simulink model "mrefrobotarm_previous_y_previous_u_previous_ref_cex_3b"  (R2018b)
settings: Solver=FixedStepAuto  StartTime=0.0  StopTime=20  RelTol=1e-3  AbsTol=1e-6
undefined symbols (not defined in the file or in its folder): cc, options
libraries: neural x462, simulink x2
(part 4 of 18)

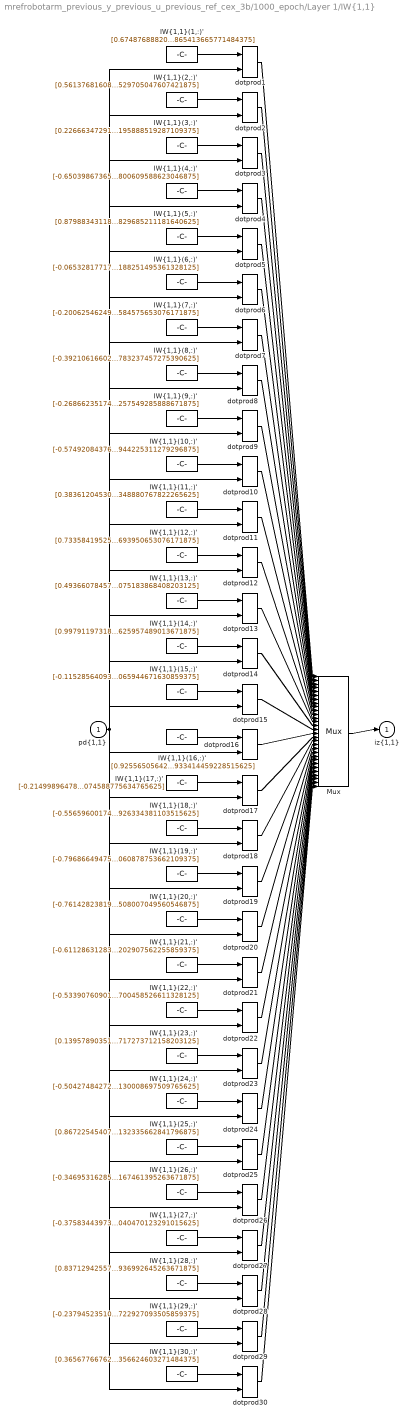
== system mrefrobotarm_previous_y_previous_u_previous_ref_cex_3b/1000_epoch/Layer 1/IW{1,1} ==
  "pd{1,1}" : Inport  PortDimensions=10
      mask Display: e = 0.06;c1 = [120 230 180]/255;c2 = ([120 230 180]+0)/(256+128);c3 = ([120 230 180]+128)/(256+128);patch([0 1 1 0],[0 0 1 1],c1);patch([0 1 1 1-e 1-e 0+e],[0 0 1 1-e 0+e 0+e],c2);patch([0 0 1 1-e 0+e 0+e],[0 1 1 1-e 1-e 0+e],c3);plot([0 1 1 0 0],[0 0 1 1 0]);
  "IW{1,1}(1,:)'" : Constant  Value=[0.67487688820245617105086921583279035985469818115234375;0.489109853240939196350467454976751469075679779052734375;-1.068845446514034680518534514703787863254547119140625;0.21467874123306529554611188359558582305908203125;1.2453232389863388984707626150338910520076751708984375;-0.485155755597752313956760872315499000251293182373046875;0.117400971307613843919170903973281383514404296875;-1.0340884350509644828974842312163673341274261474609375;2.732184740736296912899661037954501807689666748046875;4.26172786638146217086386968730948865413665771484375]
      mask Display: e = 0.06;c1 = [120 150 230]/255;c2 = ([120 150 230]+0)/383;c3 = ([120 150 230]+128)/383;patch([0 1 1 0],[0 0 1 1],c1);patch([0 1 1 1-e 1-e 0+e],[0 0 1 1-e 0+e 0+e],c2);patch([0 0 1 1-e 0+e 0+e],[0 1 1 1-e 1-e 0+e],c3);plot([0 1 1 0 0],[0 0 1 1 0]);disp('Weights');
  "IW{1,1}(10,:)'" : Constant  Value=[-0.57492084376879060148013422804069705307483673095703125;0.11469544369514152182265576129793771542608737945556640625;0.12055448748532505975905593231800594367086887359619140625;-0.55918043406571005249361405731178820133209228515625;-0.95764095097936152711781687685288488864898681640625;-1.877681983780480123868983355350792407989501953125;-4.68369972477810136979314847849309444427490234375;4.12980481084496720001197900273837149143218994140625;-1.55347300362387930050545037374831736087799072265625;-0.04197009317386261872950825591033208183944225311279296875]
      mask Display: e = 0.06;c1 = [120 150 230]/255;c2 = ([120 150 230]+0)/383;c3 = ([120 150 230]+128)/383;patch([0 1 1 0],[0 0 1 1],c1);patch([0 1 1 1-e 1-e 0+e],[0 0 1 1-e 0+e 0+e],c2);patch([0 0 1 1-e 0+e 0+e],[0 1 1 1-e 1-e 0+e],c3);plot([0 1 1 0 0],[0 0 1 1 0]);disp('Weights');
  "IW{1,1}(11,:)'" : Constant  Value=[0.383612045304692339531271727537387050688266754150390625;-0.37441834744799884493460240264539606869220733642578125;-1.572196829190865674519272943143732845783233642578125;-0.469582275713535557404298970141098834574222564697265625;-0.85236355280953490787254622773616574704647064208984375;-0.12317165432347110254340805113315582275390625;0.2987108481842801754879701547906734049320220947265625;0.52483270557119798827017120856908150017261505126953125;0.21737502294189947615876690178993158042430877685546875;0.69653814069038111345122388229356147348880767822265625]
      mask Display: e = 0.06;c1 = [120 150 230]/255;c2 = ([120 150 230]+0)/383;c3 = ([120 150 230]+128)/383;patch([0 1 1 0],[0 0 1 1],c1);patch([0 1 1 1-e 1-e 0+e],[0 0 1 1-e 0+e 0+e],c2);patch([0 0 1 1-e 0+e 0+e],[0 1 1 1-e 1-e 0+e],c3);plot([0 1 1 0 0],[0 0 1 1 0]);disp('Weights');
  "IW{1,1}(12,:)'" : Constant  Value=[0.73358419525220963652856198677909560501575469970703125;0.11073483182108510847196924942181794904172420501708984375;0.239998610252308453016922840106417424976825714111328125;1.3263748611689971657057185439043678343296051025390625;-0.383552641862259402483203984957071952521800994873046875;-0.64895639280684225269624221255071461200714111328125;0.406664060328740972760641625427524559199810028076171875;0.10576433377067527563664128820164478383958339691162109375;-0.1725196998259027891808869981105090118944644927978515625;0.86566960908073908864679424368659965693950653076171875]
      mask Display: e = 0.06;c1 = [120 150 230]/255;c2 = ([120 150 230]+0)/383;c3 = ([120 150 230]+128)/383;patch([0 1 1 0],[0 0 1 1],c1);patch([0 1 1 1-e 1-e 0+e],[0 0 1 1-e 0+e 0+e],c2);patch([0 0 1 1-e 0+e 0+e],[0 1 1 1-e 1-e 0+e],c3);plot([0 1 1 0 0],[0 0 1 1 0]);disp('Weights');
  "IW{1,1}(13,:)'" : Constant  Value=[0.493660784573921096463067215154296718537807464599609375;-0.252852678422424370641152790994965471327304840087890625;0.77470538036599745357335677908849902451038360595703125;0.00925012421792863193115152853351901285350322723388671875;0.93836282792411085384998159497627057135105133056640625;-0.52546190119467095502869824485969729721546173095703125;0.247546801452324161108009548115660436451435089111328125;-0.339457032170829953177104698625043965876102447509765625;-2.052837829371420230728517708485014736652374267578125;-0.70155465814033857174791819488746114075183868408203125]
      mask Display: e = 0.06;c1 = [120 150 230]/255;c2 = ([120 150 230]+0)/383;c3 = ([120 150 230]+128)/383;patch([0 1 1 0],[0 0 1 1],c1);patch([0 1 1 1-e 1-e 0+e],[0 0 1 1-e 0+e 0+e],c2);patch([0 0 1 1-e 0+e 0+e],[0 1 1 1-e 1-e 0+e],c3);plot([0 1 1 0 0],[0 0 1 1 0]);disp('Weights');
  "IW{1,1}(14,:)'" : Constant  Value=[0.99791197318916469161109716878854669630527496337890625;-0.9694834789619761750145698897540569305419921875;-0.341004964206196969911388805485330522060394287109375;1.132787313027051379066278968821279704570770263671875;-0.272808823384909970855005667544901371002197265625;0.283901890384503807762683891269261948764324188232421875;0.57081006863483085833621544225024990737438201904296875;-0.2053654400897696186145680030676885508000850677490234375;-0.1163006140612069250206417336812592111527919769287109375;0.2464533721904866581109416756589780561625957489013671875]
      mask Display: e = 0.06;c1 = [120 150 230]/255;c2 = ([120 150 230]+0)/383;c3 = ([120 150 230]+128)/383;patch([0 1 1 0],[0 0 1 1],c1);patch([0 1 1 1-e 1-e 0+e],[0 0 1 1-e 0+e 0+e],c2);patch([0 0 1 1-e 0+e 0+e],[0 1 1 1-e 1-e 0+e],c3);plot([0 1 1 0 0],[0 0 1 1 0]);disp('Weights');
  "IW{1,1}(15,:)'" : Constant  Value=[-0.115285640933125266283099108477472327649593353271484375;0.5697977872341686289558992939419113099575042724609375;0.62108428399830273303194871914456598460674285888671875;-0.54952679907287105276481042892555706202983856201171875;0.35326257308938957546473602633341215550899505615234375;0.4633177976030673494989287064527161419391632080078125;-0.66185527830255230785638786983327008783817291259765625;0.691823443091035716889791729045100510120391845703125;0.00067210895363132715403520212049670590204186737537384033203125;-0.239212812545204156489120350670418702065944671630859375]
      mask Display: e = 0.06;c1 = [120 150 230]/255;c2 = ([120 150 230]+0)/383;c3 = ([120 150 230]+128)/383;patch([0 1 1 0],[0 0 1 1],c1);patch([0 1 1 1-e 1-e 0+e],[0 0 1 1-e 0+e 0+e],c2);patch([0 0 1 1-e 0+e 0+e],[0 1 1 1-e 1-e 0+e],c3);plot([0 1 1 0 0],[0 0 1 1 0]);disp('Weights');
  "IW{1,1}(16,:)'" : Constant  Value=[0.92556505642418318569042412491398863494396209716796875;0.28930623759198736966169462903053499758243560791015625;0.36240767689678055063495776266790926456451416015625;-0.3168746691965560469128604381694458425045013427734375;-0.95832258235062106610513410487328656017780303955078125;-0.530791618349647276176028753980062901973724365234375;-0.9620465187669389184321744323824532330036163330078125;-0.7723827050436777863495763085666112601757049560546875;-0.021742021147157113147851958956380258314311504364013671875;-0.24232757047319053445022518644691444933414459228515625]
      mask Display: e = 0.06;c1 = [120 150 230]/255;c2 = ([120 150 230]+0)/383;c3 = ([120 150 230]+128)/383;patch([0 1 1 0],[0 0 1 1],c1);patch([0 1 1 1-e 1-e 0+e],[0 0 1 1-e 0+e 0+e],c2);patch([0 0 1 1-e 0+e 0+e],[0 1 1 1-e 1-e 0+e],c3);plot([0 1 1 0 0],[0 0 1 1 0]);disp('Weights');
  "IW{1,1}(17,:)'" : Constant  Value=[-0.214998964780564849608168742634006775915622711181640625;0.03136139918738341247905765385439735837280750274658203125;0.6519296243056051931574756963527761399745941162109375;-0.5401059522748663521696244060876779258251190185546875;0.86205331519847805399336948539712466299533843994140625;-0.51946190600488095778786146183847449719905853271484375;0.72628640014572443117657485345262102782726287841796875;-0.567247315526303363952820291160605847835540771484375;-0.750619797660048160281576201668940484523773193359375;-0.83055321633535206249376869891420938074588775634765625]
      mask Display: e = 0.06;c1 = [120 150 230]/255;c2 = ([120 150 230]+0)/383;c3 = ([120 150 230]+128)/383;patch([0 1 1 0],[0 0 1 1],c1);patch([0 1 1 1-e 1-e 0+e],[0 0 1 1-e 0+e 0+e],c2);patch([0 0 1 1-e 0+e 0+e],[0 1 1 1-e 1-e 0+e],c3);plot([0 1 1 0 0],[0 0 1 1 0]);disp('Weights');
  "IW{1,1}(18,:)'" : Constant  Value=[-0.55659600174665058158751662631402723491191864013671875;0.1838252831384339092135604687427985481917858123779296875;0.5591313930680239518977714396896772086620330810546875;-0.782611255178258691245218869880773127079010009765625;-0.90738668014734125133458064738078974187374114990234375;-1.247901387086550517580008090590126812458038330078125;0.70699009297669557216892144424491561949253082275390625;-0.07523931790047726220205248637284967117011547088623046875;-0.094213150704157921921932938857935369014739990234375;0.59139757346631383061463793637813068926334381103515625]
      mask Display: e = 0.06;c1 = [120 150 230]/255;c2 = ([120 150 230]+0)/383;c3 = ([120 150 230]+128)/383;patch([0 1 1 0],[0 0 1 1],c1);patch([0 1 1 1-e 1-e 0+e],[0 0 1 1-e 0+e 0+e],c2);patch([0 0 1 1-e 0+e 0+e],[0 1 1 1-e 1-e 0+e],c3);plot([0 1 1 0 0],[0 0 1 1 0]);disp('Weights');
  "IW{1,1}(19,:)'" : Constant  Value=[-0.79686649475483994908842078075394965708255767822265625;0.300059303789696973918665889868861995637416839599609375;0.0135495854713784426304190589007703238166868686676025390625;0.70431389745351979936316411112784408032894134521484375;0.936522954475813573793629984720610082149505615234375;-0.798693820475764315602873466559685766696929931640625;0.659356284198693298748139568488113582134246826171875;-0.451774863113715785534196811568108387291431427001953125;-0.5935337162880964800848460072302259504795074462890625;-0.329225172565789758749588145292364060878753662109375]
      mask Display: e = 0.06;c1 = [120 150 230]/255;c2 = ([120 150 230]+0)/383;c3 = ([120 150 230]+128)/383;patch([0 1 1 0],[0 0 1 1],c1);patch([0 1 1 1-e 1-e 0+e],[0 0 1 1-e 0+e 0+e],c2);patch([0 0 1 1-e 0+e 0+e],[0 1 1 1-e 1-e 0+e],c3);plot([0 1 1 0 0],[0 0 1 1 0]);disp('Weights');
  "IW{1,1}(2,:)'" : Constant  Value=[0.56137681608146972056516688098781742155551910400390625;-0.71605642152647541731624869498773477971553802490234375;0.54505402752297993362873285150271840393543243408203125;-0.93714079286020124381906271082698367536067962646484375;0.762597923999951188278600966441445052623748779296875;0.08538607921715872517420820031475159339606761932373046875;0.0313672539849252363097775742062367498874664306640625;-0.70354828725734652739021157685783691704273223876953125;0.6167387216214439416006598548847250640392303466796875;-0.6277704981014629037616714413161389529705047607421875]
      mask Display: e = 0.06;c1 = [120 150 230]/255;c2 = ([120 150 230]+0)/383;c3 = ([120 150 230]+128)/383;patch([0 1 1 0],[0 0 1 1],c1);patch([0 1 1 1-e 1-e 0+e],[0 0 1 1-e 0+e 0+e],c2);patch([0 0 1 1-e 0+e 0+e],[0 1 1 1-e 1-e 0+e],c3);plot([0 1 1 0 0],[0 0 1 1 0]);disp('Weights');
  "IW{1,1}(20,:)'" : Constant  Value=[-0.7614282381949364353346254574717022478580474853515625;0.42146161627299905116927902781753800809383392333984375;-0.81688784687210269641610693724942393600940704345703125;-0.9609461086349966318920223784516565501689910888671875;0.00095400815197363951492004474630448385141789913177490234375;0.490871455546243395939853826348553411662578582763671875;0.84805853244939710666727705756784416735172271728515625;0.54300812079479043870122723092208616435527801513671875;-0.4115204140916055575161180968279950320720672607421875;-0.306854237249814143506654318116488866508007049560546875]
      mask Display: e = 0.06;c1 = [120 150 230]/255;c2 = ([120 150 230]+0)/383;c3 = ([120 150 230]+128)/383;patch([0 1 1 0],[0 0 1 1],c1);patch([0 1 1 1-e 1-e 0+e],[0 0 1 1-e 0+e 0+e],c2);patch([0 0 1 1-e 0+e 0+e],[0 1 1 1-e 1-e 0+e],c3);plot([0 1 1 0 0],[0 0 1 1 0]);disp('Weights');
  "IW{1,1}(21,:)'" : Constant  Value=[-0.611286312839302237165384212858043611049652099609375;0.63407969352611892599469456399674527347087860107421875;0.58603475277253080921724404106498695909976959228515625;0.476103673854536335596776552847586572170257568359375;-0.00993023704667260476153245463137864135205745697021484375;0.2594575516790171842984591421554796397686004638671875;1.1155542797571424973313014561426825821399688720703125;-0.72737555296358902268138990621082484722137451171875;-0.53934483683291023492500926295178942382335662841796875;-2.2949676456640730748404166661202907562255859375]
      mask Display: e = 0.06;c1 = [120 150 230]/255;c2 = ([120 150 230]+0)/383;c3 = ([120 150 230]+128)/383;patch([0 1 1 0],[0 0 1 1],c1);patch([0 1 1 1-e 1-e 0+e],[0 0 1 1-e 0+e 0+e],c2);patch([0 0 1 1-e 0+e 0+e],[0 1 1 1-e 1-e 0+e],c3);plot([0 1 1 0 0],[0 0 1 1 0]);disp('Weights');
  "IW{1,1}(22,:)'" : Constant  Value=[-0.533907609011223360795383996446616947650909423828125;0.458913424877127218426409172025159932672977447509765625;0.1870202956799537907794928059956873767077922821044921875;-0.93941207885463706706019593184464611113071441650390625;1.002966256291259572464014127035625278949737548828125;-0.2081862916461530710332539229057147167623043060302734375;-0.56629117913395232708495541373849846422672271728515625;-1.0548815515779506046811775377136655151844024658203125;-0.0667672750543040482984480377126601524651050567626953125;0.0248600416070402681356643626031655003316700458526611328125]
      mask Display: e = 0.06;c1 = [120 150 230]/255;c2 = ([120 150 230]+0)/383;c3 = ([120 150 230]+128)/383;patch([0 1 1 0],[0 0 1 1],c1);patch([0 1 1 1-e 1-e 0+e],[0 0 1 1-e 0+e 0+e],c2);patch([0 0 1 1-e 0+e 0+e],[0 1 1 1-e 1-e 0+e],c3);plot([0 1 1 0 0],[0 0 1 1 0]);disp('Weights');
  "IW{1,1}(23,:)'" : Constant  Value=[0.1395789035139385070305451108652050606906414031982421875;-0.53570566238780192858115469789481721818447113037109375;0.295961299308874659086399105945019982755184173583984375;0.00558216036910632630585471503081862465478479862213134765625;-0.62872954655434565296445725834928452968597412109375;-0.47643791535643609247330232392414472997188568115234375;0.93956653240582266306546443956904113292694091796875;0.7882986175738897483000755528337322175502777099609375;0.655094487511215906039296896778978407382965087890625;-0.467525783216861168245515045782667584717273712158203125]
      mask Display: e = 0.06;c1 = [120 150 230]/255;c2 = ([120 150 230]+0)/383;c3 = ([120 150 230]+128)/383;patch([0 1 1 0],[0 0 1 1],c1);patch([0 1 1 1-e 1-e 0+e],[0 0 1 1-e 0+e 0+e],c2);patch([0 0 1 1-e 0+e 0+e],[0 1 1 1-e 1-e 0+e],c3);plot([0 1 1 0 0],[0 0 1 1 0]);disp('Weights');
  "IW{1,1}(24,:)'" : Constant  Value=[-0.50427484272225664430067126886569894850254058837890625;-0.2297759487395284738742162744529196061193943023681640625;0.91639348170370016344321584256249479949474334716796875;0.691749899623790742708706602570600807666778564453125;-0.439720587336256463206751732286647893488407135009765625;-0.2101612096247266470161463303156779147684574127197265625;0.209582851415682502871362657970166765153408050537109375;-1.0112001891017137200634579130564816296100616455078125;-0.93663883515621015884988764810259453952312469482421875;0.10330222853391879400675179567770101130008697509765625]
      mask Display: e = 0.06;c1 = [120 150 230]/255;c2 = ([120 150 230]+0)/383;c3 = ([120 150 230]+128)/383;patch([0 1 1 0],[0 0 1 1],c1);patch([0 1 1 1-e 1-e 0+e],[0 0 1 1-e 0+e 0+e],c2);patch([0 0 1 1-e 0+e 0+e],[0 1 1 1-e 1-e 0+e],c3);plot([0 1 1 0 0],[0 0 1 1 0]);disp('Weights');
  "IW{1,1}(25,:)'" : Constant  Value=[0.86722545407206930168086955745820887386798858642578125;0.39441717307462476060919698284124024212360382080078125;0.56122851928523520559366488669184036552906036376953125;0.82484363703543284174202199210412800312042236328125;0.323774421198204709337886697539943270385265350341796875;-0.1224445798830934573064865844571613706648349761962890625;-0.108804865459277311234842500198283232748508453369140625;0.89915240189648815150036398335942067205905914306640625;0.080636008961304461717389813202316872775554656982421875;-0.035216156921053946848854110385218518786132335662841796875]
      mask Display: e = 0.06;c1 = [120 150 230]/255;c2 = ([120 150 230]+0)/383;c3 = ([120 150 230]+128)/383;patch([0 1 1 0],[0 0 1 1],c1);patch([0 1 1 1-e 1-e 0+e],[0 0 1 1-e 0+e 0+e],c2);patch([0 0 1 1-e 0+e 0+e],[0 1 1 1-e 1-e 0+e],c3);plot([0 1 1 0 0],[0 0 1 1 0]);disp('Weights');
  "IW{1,1}(26,:)'" : Constant  Value=[-0.34695316285095711972275012158206664025783538818359375;-0.47807691883953873368540143928839825093746185302734375;-0.15820666993824084034514498853241093456745147705078125;0.94648773273035613495807183426222763955593109130859375;0.87854390005224736182043443477596156299114227294921875;0.01531186403691969961926577781241576303727924823760986328125;0.74252079132512716075353864653152413666248321533203125;-0.740147548921921583087168983183801174163818359375;1.9885517804658905394177281777956523001194000244140625;0.1849739951278592808847633932600729167461395263671875]
      mask Display: e = 0.06;c1 = [120 150 230]/255;c2 = ([120 150 230]+0)/383;c3 = ([120 150 230]+128)/383;patch([0 1 1 0],[0 0 1 1],c1);patch([0 1 1 1-e 1-e 0+e],[0 0 1 1-e 0+e 0+e],c2);patch([0 0 1 1-e 0+e 0+e],[0 1 1 1-e 1-e 0+e],c3);plot([0 1 1 0 0],[0 0 1 1 0]);disp('Weights');
  "IW{1,1}(27,:)'" : Constant  Value=[-0.375834439735718339736791904215351678431034088134765625;-0.51601512125509685358082379025290720164775848388671875;0.51906229457970864960003609667182900011539459228515625;0.254802658866700004747229968415922485291957855224609375;0.9545457694237156065497629242599941790103912353515625;-0.18793632847022478937759615291724912822246551513671875;0.64527400791439937233207047029281966388225555419921875;-0.7330021540928755019450591134955175220966339111328125;-1.3115700995600179101785442981054075062274932861328125;0.992533885729470544134755982668139040470123291015625]
      mask Display: e = 0.06;c1 = [120 150 230]/255;c2 = ([120 150 230]+0)/383;c3 = ([120 150 230]+128)/383;patch([0 1 1 0],[0 0 1 1],c1);patch([0 1 1 1-e 1-e 0+e],[0 0 1 1-e 0+e 0+e],c2);patch([0 0 1 1-e 0+e 0+e],[0 1 1 1-e 1-e 0+e],c3);plot([0 1 1 0 0],[0 0 1 1 0]);disp('Weights');
  "IW{1,1}(28,:)'" : Constant  Value=[0.8371294255751300372736523058847524225711822509765625;0.77520349715967917791914487679605372250080108642578125;0.26154071311797155718892327058711089193820953369140625;-0.46739302106909030865011800415231846272945404052734375;0.271386561162904549338037440975313074886798858642578125;-0.7082166028703091864571206315304152667522430419921875;0.67153536575519134910194907206459902226924896240234375;0.64479052144719606332046168972738087177276611328125;0.339893779477796531551803127513267099857330322265625;-1.0879156679025185905373973582754842936992645263671875]
      mask Display: e = 0.06;c1 = [120 150 230]/255;c2 = ([120 150 230]+0)/383;c3 = ([120 150 230]+128)/383;patch([0 1 1 0],[0 0 1 1],c1);patch([0 1 1 1-e 1-e 0+e],[0 0 1 1-e 0+e 0+e],c2);patch([0 0 1 1-e 0+e 0+e],[0 1 1 1-e 1-e 0+e],c3);plot([0 1 1 0 0],[0 0 1 1 0]);disp('Weights');
  "IW{1,1}(29,:)'" : Constant  Value=[-0.237945235103964203293713808307074941694736480712890625;0.38817367956647397253533426919602788984775543212890625;0.01046359712698616446779897870555942063219845294952392578125;-1.1055017083227969276748581251013092696666717529296875;0.467190762498253808754355986820883117616176605224609375;0.86723376504302496226017638036864809691905975341796875;-1.022443679265189420135584441595710813999176025390625;-0.1836511169067727433645842438636464066803455352783203125;-0.00116290070001753820770618030877585624693892896175384521484375;0.79887058034866453848366063539288006722927093505859375]
      mask Display: e = 0.06;c1 = [120 150 230]/255;c2 = ([120 150 230]+0)/383;c3 = ([120 150 230]+128)/383;patch([0 1 1 0],[0 0 1 1],c1);patch([0 1 1 1-e 1-e 0+e],[0 0 1 1-e 0+e 0+e],c2);patch([0 0 1 1-e 0+e 0+e],[0 1 1 1-e 1-e 0+e],c3);plot([0 1 1 0 0],[0 0 1 1 0]);disp('Weights');
  "IW{1,1}(3,:)'" : Constant  Value=[0.2266634729165415140794692661074805073440074920654296875;1.29135481186869061076549769495613873004913330078125;10.61884111155115562041828525252640247344970703125;33.78691572618104288494578213430941104888916015625;10.6479045294030356672010384500026702880859375;2.253192525212081687158161003026179969310760498046875;4.92810667395426538206493205507285892963409423828125;9.01681711600821955698847887106239795684814453125;0.769204381303576933959220696124248206615447998046875;7.88681873826228407864391556358896195888519287109375]
      mask Display: e = 0.06;c1 = [120 150 230]/255;c2 = ([120 150 230]+0)/383;c3 = ([120 150 230]+128)/383;patch([0 1 1 0],[0 0 1 1],c1);patch([0 1 1 1-e 1-e 0+e],[0 0 1 1-e 0+e 0+e],c2);patch([0 0 1 1-e 0+e 0+e],[0 1 1 1-e 1-e 0+e],c3);plot([0 1 1 0 0],[0 0 1 1 0]);disp('Weights');
  "IW{1,1}(30,:)'" : Constant  Value=[0.365677667625934843531609885758371092379093170166015625;-0.293570351847810606660260646094684489071369171142578125;-0.96800426625346858156007101570139639079570770263671875;0.312253548963192961718249307523365132510662078857421875;-0.35315839703492601930889804862090386450290679931640625;0.2382118836073247314377709926702664233744144439697265625;0.49575886292942550337414786554290913045406341552734375;0.1527440648261670086416330605061375536024570465087890625;-1.4390456564730078614644526169286109507083892822265625;-0.70769255391762742046779521842836402356624603271484375]
      mask Display: e = 0.06;c1 = [120 150 230]/255;c2 = ([120 150 230]+0)/383;c3 = ([120 150 230]+128)/383;patch([0 1 1 0],[0 0 1 1],c1);patch([0 1 1 1-e 1-e 0+e],[0 0 1 1-e 0+e 0+e],c2);patch([0 0 1 1-e 0+e 0+e],[0 1 1 1-e 1-e 0+e],c3);plot([0 1 1 0 0],[0 0 1 1 0]);disp('Weights');
  "IW{1,1}(4,:)'" : Constant  Value=[-0.65039867365935288834322136608534492552280426025390625;-0.6783670406823152365660689611104317009449005126953125;-0.11774102639838250616843851048543001525104045867919921875;0.71745694002003002065492864858242683112621307373046875;0.9250823925354649812646812279126606881618499755859375;-0.6098807547745719315201995414099656045436859130859375;0.203372132630537993946973074343986809253692626953125;0.14359715272293716026297261123545467853546142578125;0.5133936097644851148658062811591662466526031494140625;-0.7999467203184333907728387202951125800609588623046875]
      mask Display: e = 0.06;c1 = [120 150 230]/255;c2 = ([120 150 230]+0)/383;c3 = ([120 150 230]+128)/383;patch([0 1 1 0],[0 0 1 1],c1);patch([0 1 1 1-e 1-e 0+e],[0 0 1 1-e 0+e 0+e],c2);patch([0 0 1 1-e 0+e 0+e],[0 1 1 1-e 1-e 0+e],c3);plot([0 1 1 0 0],[0 0 1 1 0]);disp('Weights');
  "IW{1,1}(5,:)'" : Constant  Value=[0.8798834311879668579337021583341993391513824462890625;1.0257791435360463783155182682094164192676544189453125;-0.661529650792450407692513181245885789394378662109375;-0.354152587636981486252096829048241488635540008544921875;0.270117911823150980143992683224496431648731231689453125;0.286108813489685920306015987080172635614871978759765625;0.205594837916486972151375312023446895182132720947265625;-0.581814449365241070921683785854838788509368896484375;-0.9552814714234261206371456864872016012668609619140625;-0.04824437911755696806181958891102112829685211181640625]
      mask Display: e = 0.06;c1 = [120 150 230]/255;c2 = ([120 150 230]+0)/383;c3 = ([120 150 230]+128)/383;patch([0 1 1 0],[0 0 1 1],c1);patch([0 1 1 1-e 1-e 0+e],[0 0 1 1-e 0+e 0+e],c2);patch([0 0 1 1-e 0+e 0+e],[0 1 1 1-e 1-e 0+e],c3);plot([0 1 1 0 0],[0 0 1 1 0]);disp('Weights');
  "IW{1,1}(6,:)'" : Constant  Value=[-0.065328177178999136121007040856056846678256988525390625;-0.88750616201524945569900637565297074615955352783203125;0.58917923699212437771421946308691985905170440673828125;-0.273117847684619940995531806038343347609043121337890625;0.75810672187664795984574084286577999591827392578125;0.347805132221497448341551717021502554416656494140625;0.79653455491702995772129725082777440547943115234375;0.526683299581100161645963453338481485843658447265625;-3.8703305558273886077813585870899260044097900390625;-4.3590551354574689213450255920179188251495361328125]
      mask Display: e = 0.06;c1 = [120 150 230]/255;c2 = ([120 150 230]+0)/383;c3 = ([120 150 230]+128)/383;patch([0 1 1 0],[0 0 1 1],c1);patch([0 1 1 1-e 1-e 0+e],[0 0 1 1-e 0+e 0+e],c2);patch([0 0 1 1-e 0+e 0+e],[0 1 1 1-e 1-e 0+e],c3);plot([0 1 1 0 0],[0 0 1 1 0]);disp('Weights');
  "IW{1,1}(7,:)'" : Constant  Value=[-0.2006254624908041239716993686670321039855480194091796875;0.1643201458624764244031979387727915309369564056396484375;0.86209723696338269594008352214586921036243438720703125;0.4482801075555620240464804737712256610393524169921875;0.0526937616399284214363518685786402784287929534912109375;-0.90580581566849593944112939425394870340824127197265625;-0.59732039694270344654114524018950760364532470703125;-0.84912806806211638122050544552621431648731231689453125;-0.53496892663123796207713667172356508672237396240234375;1.540370790189356409172205530921928584575653076171875]
      mask Display: e = 0.06;c1 = [120 150 230]/255;c2 = ([120 150 230]+0)/383;c3 = ([120 150 230]+128)/383;patch([0 1 1 0],[0 0 1 1],c1);patch([0 1 1 1-e 1-e 0+e],[0 0 1 1-e 0+e 0+e],c2);patch([0 0 1 1-e 0+e 0+e],[0 1 1 1-e 1-e 0+e],c3);plot([0 1 1 0 0],[0 0 1 1 0]);disp('Weights');
  "IW{1,1}(8,:)'" : Constant  Value=[-0.3921061660263849280028125576791353523731231689453125;1.02406515222817073862415782059542834758758544921875;-0.51538656004868477200631105006323195993900299072265625;-0.9058835091524006788432643588748760521411895751953125;-0.38295393174394332103105398346087895333766937255859375;0.3773318218134151802445330758928321301937103271484375;0.10090741553520576889724225111422128975391387939453125;1.23323414571400302719439423526637256145477294921875;0.44289852642448845898570652934722602367401123046875;2.844151440413919207372828168445266783237457275390625]
      mask Display: e = 0.06;c1 = [120 150 230]/255;c2 = ([120 150 230]+0)/383;c3 = ([120 150 230]+128)/383;patch([0 1 1 0],[0 0 1 1],c1);patch([0 1 1 1-e 1-e 0+e],[0 0 1 1-e 0+e 0+e],c2);patch([0 0 1 1-e 0+e 0+e],[0 1 1 1-e 1-e 0+e],c3);plot([0 1 1 0 0],[0 0 1 1 0]);disp('Weights');
  "IW{1,1}(9,:)'" : Constant  Value=[-0.268662351749143823997911795231630094349384307861328125;-0.349751792894843760439727020639111287891864776611328125;0.2485298328135374656966405382263474166393280029296875;-0.248759668053308902191389506697305478155612945556640625;-0.79872614553731191566754432642483152449131011962890625;0.262666930256094222073670607642270624637603759765625;-0.90291238898472114815518807517946697771549224853515625;0.5199527483089030344132197569706477224826812744140625;-0.78256104079507060600207069001044146716594696044921875;-1.208048438166343441224626076291315257549285888671875]
      mask Display: e = 0.06;c1 = [120 150 230]/255;c2 = ([120 150 230]+0)/383;c3 = ([120 150 230]+128)/383;patch([0 1 1 0],[0 0 1 1],c1);patch([0 1 1 1-e 1-e 0+e],[0 0 1 1-e 0+e 0+e],c2);patch([0 0 1 1-e 0+e 0+e],[0 1 1 1-e 1-e 0+e],c3);plot([0 1 1 0 0],[0 0 1 1 0]);disp('Weights');
  Mux : Mux  Inputs=30
      mask Display: e = 0.06;c1 = [120 150 230]/255;c2 = ([120 150 230]+0)/383;c3 = ([120 150 230]+128)/383;patch([0 1 1 0],[0 0 1 1],c1);patch([0 1 1 1-e 1-e 0+e],[0 0 1 1-e 0+e 0+e],c2);patch([0 0 1 1-e 0+e 0+e],[0 1 1 1-e 1-e 0+e],c3);plot([0 1 1 0 0],[0 0 1 1 0]);disp('Mux');
  dotprod{1..30} (30 alike) : neural/Weight Functions/dotprod
  "iz{1,1}" : Outport
      mask Display: e = 0.06;c1 = [120 230 180]/255;c2 = ([120 230 180]+0)/(256+128);c3 = ([120 230 180]+128)/(256+128);patch([0 1 1 0],[0 0 1 1],c1);patch([0 1 1 1-e 1-e 0+e],[0 0 1 1-e 0+e 0+e],c2);patch([0 0 1 1-e 0+e 0+e],[0 1 1 1-e 1-e 0+e],c3);plot([0 1 1 0 0],[0 0 1 1 0]);
  wires:
  "IW{1,1}(1,:)'"/1 -> dotprod1/1
  "pd{1,1}"/1 -> dotprod1/2, dotprod2/2, dotprod3/2, dotprod4/2, dotprod5/2, dotprod6/2, dotprod7/2, dotprod8/2, dotprod9/2, dotprod10/2, dotprod11/2, dotprod12/2, dotprod13/2, dotprod14/2, dotprod15/2, dotprod16/2, dotprod17/2, dotprod18/2, dotprod19/2, dotprod20/2, dotprod21/2, dotprod22/2, dotprod23/2, dotprod24/2, dotprod25/2, dotprod26/2, dotprod27/2, dotprod28/2, dotprod29/2, dotprod30/2
  dotprod1/1 -> Mux/1
  "IW{1,1}(2,:)'"/1 -> dotprod2/1
  dotprod2/1 -> Mux/2
  "IW{1,1}(3,:)'"/1 -> dotprod3/1
  dotprod3/1 -> Mux/3
  "IW{1,1}(4,:)'"/1 -> dotprod4/1
  dotprod4/1 -> Mux/4
  "IW{1,1}(5,:)'"/1 -> dotprod5/1
  dotprod5/1 -> Mux/5
  "IW{1,1}(6,:)'"/1 -> dotprod6/1
  dotprod6/1 -> Mux/6
  "IW{1,1}(7,:)'"/1 -> dotprod7/1
  dotprod7/1 -> Mux/7
  "IW{1,1}(8,:)'"/1 -> dotprod8/1
  dotprod8/1 -> Mux/8
  "IW{1,1}(9,:)'"/1 -> dotprod9/1
  dotprod9/1 -> Mux/9
  "IW{1,1}(10,:)'"/1 -> dotprod10/1
  dotprod10/1 -> Mux/10
  "IW{1,1}(11,:)'"/1 -> dotprod11/1
  dotprod11/1 -> Mux/11
  "IW{1,1}(12,:)'"/1 -> dotprod12/1
  dotprod12/1 -> Mux/12
  "IW{1,1}(13,:)'"/1 -> dotprod13/1
  dotprod13/1 -> Mux/13
  "IW{1,1}(14,:)'"/1 -> dotprod14/1
  dotprod14/1 -> Mux/14
  "IW{1,1}(15,:)'"/1 -> dotprod15/1
  dotprod15/1 -> Mux/15
  "IW{1,1}(16,:)'"/1 -> dotprod16/1
  dotprod16/1 -> Mux/16
  "IW{1,1}(17,:)'"/1 -> dotprod17/1
  dotprod17/1 -> Mux/17
  "IW{1,1}(18,:)'"/1 -> dotprod18/1
  dotprod18/1 -> Mux/18
  "IW{1,1}(19,:)'"/1 -> dotprod19/1
  dotprod19/1 -> Mux/19
  "IW{1,1}(20,:)'"/1 -> dotprod20/1
  dotprod20/1 -> Mux/20
  "IW{1,1}(21,:)'"/1 -> dotprod21/1
  dotprod21/1 -> Mux/21
  "IW{1,1}(22,:)'"/1 -> dotprod22/1
  dotprod22/1 -> Mux/22
  "IW{1,1}(23,:)'"/1 -> dotprod23/1
  dotprod23/1 -> Mux/23
  "IW{1,1}(24,:)'"/1 -> dotprod24/1
  dotprod24/1 -> Mux/24
  "IW{1,1}(25,:)'"/1 -> dotprod25/1
  dotprod25/1 -> Mux/25
  "IW{1,1}(26,:)'"/1 -> dotprod26/1
  dotprod26/1 -> Mux/26
  "IW{1,1}(27,:)'"/1 -> dotprod27/1
  dotprod27/1 -> Mux/27
  "IW{1,1}(28,:)'"/1 -> dotprod28/1
  dotprod28/1 -> Mux/28
  "IW{1,1}(29,:)'"/1 -> dotprod29/1
  dotprod29/1 -> Mux/29
  "IW{1,1}(30,:)'"/1 -> dotprod30/1
  dotprod30/1 -> Mux/30
  Mux/1 -> "iz{1,1}"/1

== system mrefrobotarm_previous_y_previous_u_previous_ref_cex_3b/1000_epoch/Layer 2/Delays 1 ==
  "p{2}" : Inport  PortDimensions=30
      mask Display: e = 0.06;c1 = [120 230 180]/255;c2 = ([120 230 180]+0)/(256+128);c3 = ([120 230 180]+128)/(256+128);patch([0 1 1 0],[0 0 1 1],c1);patch([0 1 1 1-e 1-e 0+e],[0 0 1 1-e 0+e 0+e],c2);patch([0 0 1 1-e 0+e 0+e],[0 1 1 1-e 1-e 0+e],c3);plot([0 1 1 0 0],[0 0 1 1 0]);
  mux : Mux  Inputs=1
      mask Display: e = 0.06;c1 = [120 150 230]/255;c2 = ([120 150 230]+0)/383;c3 = ([120 150 230]+128)/383;patch([0 1 1 0],[0 0 1 1],c1);patch([0 1 1 1-e 1-e 0+e],[0 0 1 1-e 0+e 0+e],c2);patch([0 0 1 1-e 0+e 0+e],[0 1 1 1-e 1-e 0+e],c3);plot([0 1 1 0 0],[0 0 1 1 0]);disp('Mux')
  "pd{2,1}" : Outport
      mask Display: e = 0.06;c1 = [120 230 180]/255;c2 = ([120 230 180]+0)/(256+128);c3 = ([120 230 180]+128)/(256+128);patch([0 1 1 0],[0 0 1 1],c1);patch([0 1 1 1-e 1-e 0+e],[0 0 1 1-e 0+e 0+e],c2);patch([0 0 1 1-e 0+e 0+e],[0 1 1 1-e 1-e 0+e],c3);plot([0 1 1 0 0],[0 0 1 1 0]);
  wires:
  "p{2}"/1 -> mux/1
  mux/1 -> "pd{2,1}"/1
